simulink model "ObservadorMotorDC"  (R2020b)
settings: Solver=VariableStepAuto  StartTime=0.0  StopTime=10.0  RelTol=1e-3
libraries: fl_lib x6, nesl_utility x4, ee_lib x1
settings Model: Creator=petir  LastModifiedBy=petir

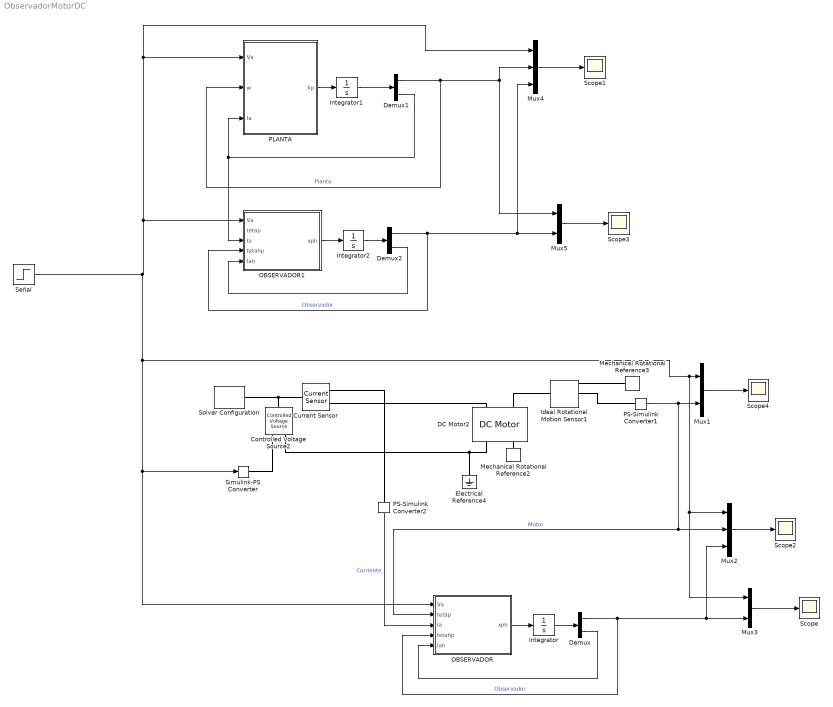
== system ObservadorMotorDC ==
  Controlled Voltage Source2 : fl_lib/Electrical/Electrical Sources/Controlled Voltage Source
  Current Sensor : fl_lib/Electrical/Electrical Sensors/Current Sensor
  DC Motor2 : ee_lib/Electromechanical/Brushed Motors/DC Motor  field_option=ee.enum.field_option.pm  Rf=100 Ohm  Lf=1 H  Laf=0.15 H  If0=0 A  parameterization=ee.enum.dcparam_option.circuit_param  Ra=8.3 Ohm  La=1.51e-3 H  emf_or_torque=ee.enum.emf_or_torque.ki  Kv=0.0879 V/(rad/s)  Ki=0.0879 N*m/A  T_stall=0.24e-3 N*m  w_max=19100 rpm  w_rated=15000 rpm  P_rated=0.08 W  V_rated=1.5 V  J=80.7e-6 kg*m^2  lam_param=ee.enum.lam_param.damping  lam=14.41e-6 N*m/(rad/s)  i_noload=0 A  V_i_noload=1.5 V  speed0=0 rpm  enable_fault_armature=ee.enum.faults.faultEnable.no  rev_faulted=1 / 3  G_faulted_armature=1e-5 S  fault_trigger_armature=ee.enum.faults.faultTrigger.temporal  t_fault_armature=1 s  max_permissible_current_armature=inf A  t_fail_on_current_armature=1 s  enable_fault_field=ee.enum.faults.faultEnable.no  G_faulted_field=1e-5 S  fault_trigger_field=ee.enum.faults.faultTrigger.temporal  t_fault_field=1 s  max_permissible_current_field=inf A  t_fail_on_current_field=1 s  fault_action=ee.enum.faults.faultAction.none  alpha=3.93e-3 1/K  Tmeas=25 degC  thermal_mass=100 J/K  initial_temperature=25 degC
  Demux : Demux  Outputs=2
  Demux1 : Demux  Outputs=2
  Demux2 : Demux  Outputs=2
  Electrical Reference4 : fl_lib/Electrical/Electrical Elements/Electrical Reference
  Ideal Rotational Motion Sensor1 : fl_lib/Mechanical/Mechanical Sensors/Ideal Rotational Motion Sensor  wrap_angle=simscape.enum.onoff.off  offset=0 rad
  Integrator : Integrator
  Integrator1 : Integrator
  Integrator2 : Integrator
  Mechanical Rotational Reference2 : fl_lib/Mechanical/Rotational Elements/Mechanical Rotational Reference
  Mechanical Rotational Reference3 : fl_lib/Mechanical/Rotational Elements/Mechanical Rotational Reference
  Mux1 : Mux  Inputs=2
  Mux2 : Mux  Inputs=3
  Mux3 : Mux  Inputs=2
  Mux4 : Mux  Inputs=3
  Mux5 : Mux  Inputs=2
  OBSERVADOR : MATLAB Function  TreatAsAtomicUnit=on
  OBSERVADOR1 : MATLAB Function  TreatAsAtomicUnit=on
  PLANTA : MATLAB Function  TreatAsAtomicUnit=on
  PS-Simulink Converter1 : nesl_utility/PS-Simulink Converter  PhysicalDomain=network_engine_domain  SubClassName=ps_output  LeftPortType=input  RightPortType=output  PseudoPeriodic=off  Frequencies=[]  Unit=inherit  AffineConversion=off
  PS-Simulink Converter2 : nesl_utility/PS-Simulink Converter  PhysicalDomain=network_engine_domain  SubClassName=ps_output  LeftPortType=input  RightPortType=output  PseudoPeriodic=off  Frequencies=[]  Unit=inherit  AffineConversion=off
  Scope{,1..4} (5 alike) : Scope
  Señal : Step  After=pi/2  SampleTime=0
  Simulink-PS Converter : nesl_utility/Simulink-PS Converter  PhysicalDomain=network_engine_domain  SubClassName=ps_input  LeftPortType=input  RightPortType=output  PseudoPeriodic=off  Frequencies=[]  NoiseDistribution=none  NoiseParameters=[]  Unit=1  AffineConversion=off  FilteringAndDerivatives=provide  SimscapeFilterOrder=1  InputFilterTimeConstant=0.001  UdotUserProvided=0
  Solver Configuration : nesl_utility/Solver Configuration  PhysicalDomain=network_engine_domain  SubClassName=solver  LeftPortType=input  RightPortType=generic  Tones=[]  Harmonics=[]  SimulateNoise=off  Profile=off  UseLocalSampling=off  EnableSwitchedLinearOptims=on  FrequencyDomain=off  UseCCode=off  RelTol=0.001  AbsTol=1e-06  MinStep=1e-09  ToWorkspace=off  RevertToSquareIcSolve=off  NumHomotopyIterations=100  PhasorMode=off  PhasorModeNumHarmonics=1  DoDC=off  ResidualTolerance=1e-09  UseLocalSolver=off  LocalSolverChoice=NE_BACKWARD_EULER_ADVANCER  LocalSolverSampleTime=0.001  DoFixedCost=off  MaxNonlinIter=3  MaxModeIter=2  ComputeImpulses=off  ImpulseIterations=2  LinearAlgebra=auto  EquationFormulation=NE_TIME_EF  DelaysMemoryBudget=1024  AutomaticFiltering=on  FilteringTimeConstant=0.001  PartitionStorageMethod=AS_NEEDED  PartitionMemoryBudget=1024  PartitionMethod=ROBUST
  wires:
  Integrator/1 -> Demux/1
  Demux/1 -> Mux2/3, Mux3/2, OBSERVADOR/4(tetahp)  "Observador"
  Mux2/1 -> Scope2/1
  Demux/2 -> OBSERVADOR/5(Iah)
  Mux3/1 -> Scope/1
  PS-Simulink Converter1/1 -> Mux1/2, OBSERVADOR/2(tetap), Mux2/2  "Motor"
  Mux1/1 -> Scope4/1
  PS-Simulink Converter2/1 -> OBSERVADOR/3(Ia)  "Corriente"
  OBSERVADOR/1(xph) -> Integrator/1
  PLANTA/1(Xp) -> Integrator1/1
  Integrator1/1 -> Demux1/1
  Demux1/2 -> PLANTA/3(Ia), OBSERVADOR1/3(Ia)
  Mux4/1 -> Scope1/1
  Señal/1 -> OBSERVADOR1/1(Va), Mux4/1, PLANTA/1(Va), Simulink-PS Converter/1, OBSERVADOR/1(Va), Mux3/1, Mux2/1, Mux1/1
  OBSERVADOR1/1(xph) -> Integrator2/1
  Mux5/1 -> Scope3/1
  Demux1/1 -> PLANTA/2(w), Mux5/1, Mux4/2  "Planta"
  Integrator2/1 -> Demux2/1
  Demux2/1 -> Mux4/3, Mux5/2, OBSERVADOR1/4(tetahp)  "Observador"
  Demux2/2 -> OBSERVADOR1/5(Iah)
  connections:
  Electrical Reference4/LConn1 -- Controlled Voltage Source2/RConn2 -- DC Motor2/RConn1
  Controlled Voltage Source2/LConn1 -- Solver Configuration/RConn1 -- Current Sensor/LConn1
  PS-Simulink Converter1/LConn1 -- Ideal Rotational Motion Sensor1/RConn2
  Simulink-PS Converter/RConn1 -- Controlled Voltage Source2/RConn1
  PS-Simulink Converter2/LConn1 -- Current Sensor/RConn1
  Current Sensor/RConn2 -- DC Motor2/LConn1
  DC Motor2/LConn2 -- Ideal Rotational Motion Sensor1/LConn1
  Ideal Rotational Motion Sensor1/RConn1 -- Mechanical Rotational Reference3/LConn1
  DC Motor2/RConn2 -- Mechanical Rotational Reference2/LConn1

== matlab function ObservadorMotorDC/PLANTA ==
  data: Va input; Xp output; w input; Ia input
function Xp = fcn(Va, w, Ia)
% Parámetros
Ra = 8.3;
Ke = 0.0879;
Ki = 0.0879;
J = 80.7e-6;
B = 14.41e-6;
TL = 0.1*0; % TL nulo

La = 1.51e-3;

% tetapp = Ki / (J * Ra) * Va - Ki * Ke / (J * Ra) * tetap - B / J * tetap - 1 / J * TL;
wp = (Ki / J) * Ia - B / J * w - 1 / J * TL;
Iap = 1 / La * Va - Ra / La * Ia - Ke / La * w;

Xp = [wp, Iap];

== matlab function ObservadorMotorDC/OBSERVADOR ==
  data: Va input; xph output; tetap input; Ia input; tetahp input; Iah input
function xph = fcn(Va, tetap, Ia, tetahp, Iah)
% Parámetros
Ra = 8.3;
La = 1.51e-3;
Ke = 0.0879;
Ki = 0.0879;
J = 80.7e-6;
B = 14.41e-6;

A = [-B / J, Ki / J; -Ke/La, -Ra / La];
B_mat = [0; 1 / La];
C = [0, 1];

x = [tetap; Ia];
xh = [tetahp; Iah];

y = C * x;
yh = C * xh;

K = [19.8214; 96.8214];
% K = [6.18*1000; -7360];

% xph = Axh + Bu + k(y-yh)
xph = A * xh + B_mat * Va + K * (y - yh);

== matlab function ObservadorMotorDC/OBSERVADOR1 ==
  data: Va input; xph output; tetap input; Ia input; tetahp input; Iah input
function xph = fcn(Va, tetap, Ia, tetahp, Iah)
% Parámetros
Ra = 8.3;
La = 1.51e-3;
Ke = 0.0879;
Ki = 0.0879;
J = 80.7e-6;
B = 14.41e-6;

A = [-B / J, Ki / J; -Ke/La, -Ra / La];
B_mat = [0; 1 / La];
C = [0, 1];

x = [tetap; Ia];
xh = [tetahp; Iah];

y = C * x;
yh = C * xh;

K = [19.8214; 96.8214];
% K = [6.18*1000; -7360];

% xph = Axh + Bu + k(y-yh)
xph = A * xh + B_mat * Va + K * (y - yh);
